simulink model "x52pro_HOTAS"  (R2019b)
settings: Solver=FixedStepDiscrete  StartTime=0.0  StopTime=inf  FixedStep=0.1  RelTol=1e-3
settings Model: EnablePacing=on  Creator=dimas  LastModifiedBy=dimas

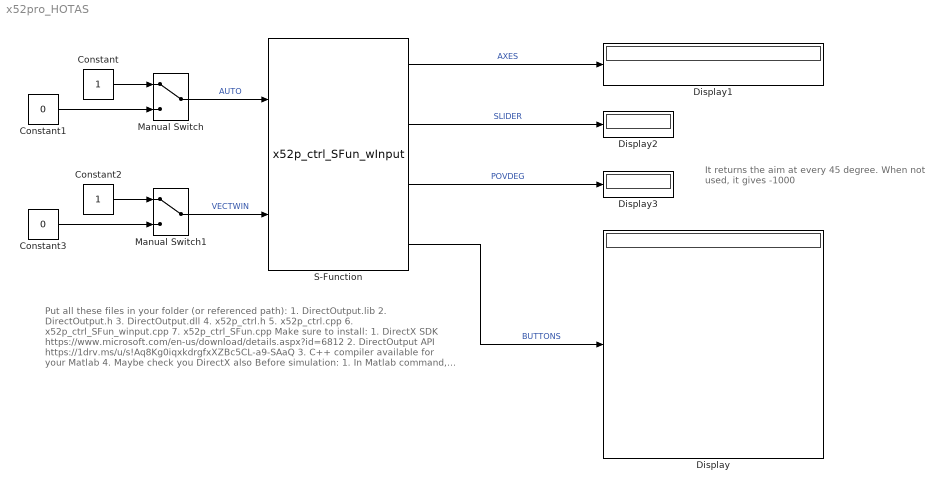
== system x52pro_HOTAS ==
  note: It returns the aim at every 45 degree.
      | When not used, it gives -1000
  note: Put all these files in your folder (or referenced path):
      |
      | 1. DirectOutput.lib
      | 2. DirectOutput.h
      | 3. DirectOutput.dll
      | 4. x52p_ctrl.h
      | 5. x52p_ctrl.cpp
      | 6. x52p_ctrl_SFun_winput.cpp
      | 7. x52p_ctrl_SFun.cpp
      |
      | Make sure to install:
      | 1. DirectX SDK
      |     https://www.microsoft.com/en-us/download/details.aspx?id=6812
      | 2. DirectOutput API
      |     https://1drv.ms/u/s!Aq8Kg0iqxkdrgfxXZBc5CL-a9-SAaQ
      | 3. C++ compiler available for your Matlab
      | 4. Maybe check you DirectX also
      |
      | Before simulation:
      | 1. In Matlab command, do mex -setup and choose the appropriate
      |     C++ compiler.
      | 2. Then compile by mex x52p_ctrl_SFun_wInput.cpp or
      |     mex x52p_ctrl_SFun.cpp, whichever you want to use.
      | 3. Double click the block, and put either x52p_ctrl_SFun_wInput or
      |     x52p_ctrl_SFun in the S-function name.
      | 4. Put 0 (the default Joystick ID) in the S-function parameters.
      | 5. In the Simulink, in the Debug tab, update the model.
      | 6. Adjust the input port accordingly (x52p_ctrl_SFun_wInput needs
      |    one input signal).
      | 7. Have fun.
      |
      | Osaka University: Dimas M. Rachman, 2022.
  Constant : Constant
  Constant1 : Constant  Value=0
  Constant2 : Constant
  Constant3 : Constant  Value=0
  Display{,1..3} (4 alike) : Display
  Manual Switch : ManualSwitch
  Manual Switch1 : ManualSwitch
  S-Function : S-Function  FunctionName=x52p_ctrl_SFun_wInput  Parameters=0  SFunctionDeploymentMode=off  EnableBusSupport=off
  wires:
  S-Function/4 -> Display/1  "BUTTONS"
  S-Function/1 -> Display1/1  "AXES"
  S-Function/2 -> Display2/1  "SLIDER"
  S-Function/3 -> Display3/1  "POVDEG"
  Constant/1 -> Manual Switch/1
  Constant1/1 -> Manual Switch/2
  Constant2/1 -> Manual Switch1/1
  Constant3/1 -> Manual Switch1/2
  Manual Switch/1 -> S-Function/1  "AUTO"
  Manual Switch1/1 -> S-Function/2  "VECTWIN"
